simulink model "DK_KGTT"  (R2018a)
settings: Solver=VariableStepAuto  StartTime=0.0  StopTime=10.0  RelTol=1e-3
libraries: simulink x3
settings Model: Creator=dtan  LastModifiedBy=dtan

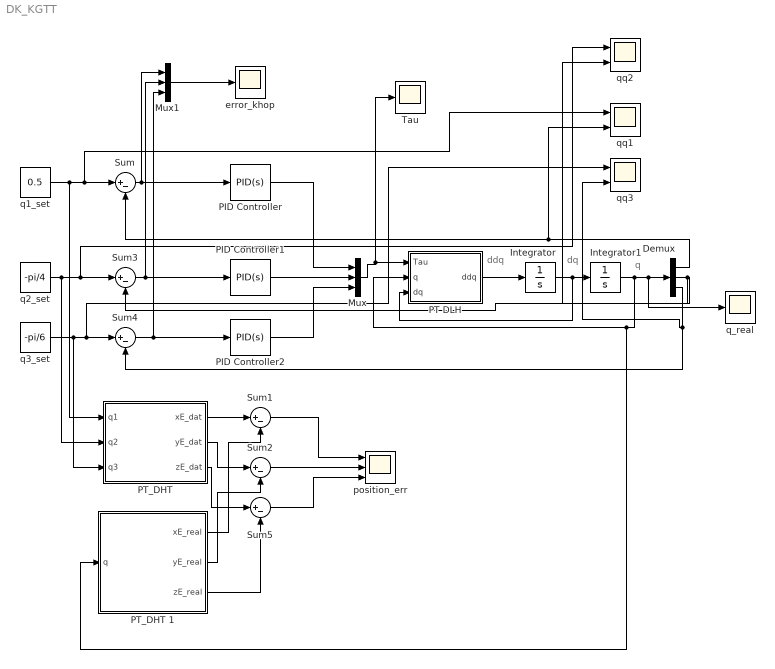
== system DK_KGTT ==
  note: q
  note: dq
  note: ddq
  Demux : Demux  Outputs=3
  Integrator : Integrator
  Integrator1 : Integrator
  Mux : Mux  Inputs=3
  Mux1 : Mux  Inputs=3
  PID Controller : simulink/Continuous/PID Controller  Controller=PID  TimeDomain=Continuous-time  SampleTime=-1  IntegratorMethod=Forward Euler  FilterMethod=Forward Euler  Form=Parallel  UseFilter=on  ControllerParametersSource=internal  P=50  I=30  D=10  N=100  InitialConditionSource=internal  InitialConditionForIntegrator=0  InitialConditionForFilter=0  ExternalReset=none  LimitOutput=off  UpperSaturationLimit=inf  LowerSaturationLimit=-inf  LinearizeAsGain=on  AntiWindupMode=none  Kb=1  TrackingMode=off  Kt=1  PParamMin=[]  PParamMax=[]  IParamMin=[]  IParamMax=[]  DParamMin=[]  DParamMax=[]  NParamMin=[]  NParamMax=[]  KbParamMin=[]  KbParamMax=[]  KtParamMin=[]  KtParamMax=[]  POutMin=[]  POutMax=[]  IOutMin=[]  IOutMax=[]  DOutMin=[]  DOutMax=[]  NOutMin=[]  NOutMax=[]  KbOutMin=[]  KbOutMax=[]  KtOutMin=[]  KtOutMax=[]  IntegratorOutMin=[]  IntegratorOutMax=[]  FilterOutMin=[]  FilterOutMax=[]  SumOutMin=[]  SumOutMax=[]  SumI1OutMin=[]  SumI1OutMax=[]  SumI2OutMin=[]  SumI2OutMax=[]  SumI3OutMin=[]  SumI3OutMax=[]  SumDOutMin=[]  SumDOutMax=[]  SaturationOutMin=[]  SaturationOutMax=[]  IntegratorContinuousStateAttributes=''  IntegratorStateMustResolveToSignalObject=off  IntegratorRTWStateStorageClass=Auto  FilterContinuousStateAttributes=''  FilterStateMustResolveToSignalObject=off  FilterRTWStateStorageClass=Auto  DifferentiatorICPrevScaledInput=0  DifferentiatorOutMin=[]  DifferentiatorOutMax=[]  FilterDiffOutCoefMin=[]  FilterDiffOutCoefMax=[]  SumDenOutMin=[]  SumDenOutMax=[]  SumNumOutMin=[]  SumNumOutMax=[]  ReciprocalOutMin=[]  ReciprocalOutMax=[]  DivideOutMin=[]  DivideOutMax=[]  TunerSelectOption=Transfer Function Based (PID Tuner App)
  PID Controller1 : simulink/Continuous/PID Controller  Controller=PID  TimeDomain=Continuous-time  SampleTime=-1  IntegratorMethod=Forward Euler  FilterMethod=Forward Euler  Form=Parallel  UseFilter=on  ControllerParametersSource=internal  P=20  I=0.2  D=0.8  N=100  InitialConditionSource=internal  InitialConditionForIntegrator=0  InitialConditionForFilter=0  ExternalReset=none  LimitOutput=off  UpperSaturationLimit=inf  LowerSaturationLimit=-inf  LinearizeAsGain=on  AntiWindupMode=none  Kb=1  TrackingMode=off  Kt=1  PParamMin=[]  PParamMax=[]  IParamMin=[]  IParamMax=[]  DParamMin=[]  DParamMax=[]  NParamMin=[]  NParamMax=[]  KbParamMin=[]  KbParamMax=[]  KtParamMin=[]  KtParamMax=[]  POutMin=[]  POutMax=[]  IOutMin=[]  IOutMax=[]  DOutMin=[]  DOutMax=[]  NOutMin=[]  NOutMax=[]  KbOutMin=[]  KbOutMax=[]  KtOutMin=[]  KtOutMax=[]  IntegratorOutMin=[]  IntegratorOutMax=[]  FilterOutMin=[]  FilterOutMax=[]  SumOutMin=[]  SumOutMax=[]  SumI1OutMin=[]  SumI1OutMax=[]  SumI2OutMin=[]  SumI2OutMax=[]  SumI3OutMin=[]  SumI3OutMax=[]  SumDOutMin=[]  SumDOutMax=[]  SaturationOutMin=[]  SaturationOutMax=[]  IntegratorContinuousStateAttributes=''  IntegratorStateMustResolveToSignalObject=off  IntegratorRTWStateStorageClass=Auto  FilterContinuousStateAttributes=''  FilterStateMustResolveToSignalObject=off  FilterRTWStateStorageClass=Auto  DifferentiatorICPrevScaledInput=0  DifferentiatorOutMin=[]  DifferentiatorOutMax=[]  FilterDiffOutCoefMin=[]  FilterDiffOutCoefMax=[]  SumDenOutMin=[]  SumDenOutMax=[]  SumNumOutMin=[]  SumNumOutMax=[]  ReciprocalOutMin=[]  ReciprocalOutMax=[]  DivideOutMin=[]  DivideOutMax=[]  TunerSelectOption=Transfer Function Based (PID Tuner App)
  PID Controller2 : simulink/Continuous/PID Controller  Controller=PID  TimeDomain=Continuous-time  SampleTime=-1  IntegratorMethod=Forward Euler  FilterMethod=Forward Euler  Form=Parallel  UseFilter=on  ControllerParametersSource=internal  P=50  I=30  D=10  N=100  InitialConditionSource=internal  InitialConditionForIntegrator=0  InitialConditionForFilter=0  ExternalReset=none  LimitOutput=off  UpperSaturationLimit=inf  LowerSaturationLimit=-inf  LinearizeAsGain=on  AntiWindupMode=none  Kb=1  TrackingMode=off  Kt=1  PParamMin=[]  PParamMax=[]  IParamMin=[]  IParamMax=[]  DParamMin=[]  DParamMax=[]  NParamMin=[]  NParamMax=[]  KbParamMin=[]  KbParamMax=[]  KtParamMin=[]  KtParamMax=[]  POutMin=[]  POutMax=[]  IOutMin=[]  IOutMax=[]  DOutMin=[]  DOutMax=[]  NOutMin=[]  NOutMax=[]  KbOutMin=[]  KbOutMax=[]  KtOutMin=[]  KtOutMax=[]  IntegratorOutMin=[]  IntegratorOutMax=[]  FilterOutMin=[]  FilterOutMax=[]  SumOutMin=[]  SumOutMax=[]  SumI1OutMin=[]  SumI1OutMax=[]  SumI2OutMin=[]  SumI2OutMax=[]  SumI3OutMin=[]  SumI3OutMax=[]  SumDOutMin=[]  SumDOutMax=[]  SaturationOutMin=[]  SaturationOutMax=[]  IntegratorContinuousStateAttributes=''  IntegratorStateMustResolveToSignalObject=off  IntegratorRTWStateStorageClass=Auto  FilterContinuousStateAttributes=''  FilterStateMustResolveToSignalObject=off  FilterRTWStateStorageClass=Auto  DifferentiatorICPrevScaledInput=0  DifferentiatorOutMin=[]  DifferentiatorOutMax=[]  FilterDiffOutCoefMin=[]  FilterDiffOutCoefMax=[]  SumDenOutMin=[]  SumDenOutMax=[]  SumNumOutMin=[]  SumNumOutMax=[]  ReciprocalOutMin=[]  ReciprocalOutMax=[]  DivideOutMin=[]  DivideOutMax=[]  TunerSelectOption=Transfer Function Based (PID Tuner App)
  PT DLH : MATLAB Function  TreatAsAtomicUnit=on
  "PT_DHT " : MATLAB Function  TreatAsAtomicUnit=on
  PT_DHT 1 : MATLAB Function  TreatAsAtomicUnit=on
  Sum{,1..5} (6 alike) : Sum  Inputs=|+-
  "Tau " : Scope
  "error_khop " : Scope
  position_err : Scope  NumInputPorts=3
  "q1_set " : Constant  Value=0.5
  q2_set : Constant  Value=-pi/4
  "q3_set " : Constant  Value=-pi/6
  "q_real " : Scope
  qq1 : Scope  NumInputPorts=2
  qq2 : Scope  NumInputPorts=2
  qq3 : Scope  NumInputPorts=2
  wires:
  Sum3/1 -> Mux1/2, PID Controller1/1
  PID Controller/1 -> Mux/1
  Demux/3 -> qq3/2, Sum4/2
  Demux/2 -> qq2/2, Sum3/2
  Mux/1 -> "Tau "/1, PT DLH/1(Tau)
  q2_set/1 -> "PT_DHT "/2(q2), qq2/1, Sum3/1
  Integrator1/1 -> "q_real "/1, Demux/1, PT_DHT 1/1(q), PT DLH/2(q)
  PID Controller1/1 -> Mux/2
  Integrator/1 -> PT DLH/3(dq), Integrator1/1
  "q1_set "/1 -> "PT_DHT "/1(q1), qq1/1, Sum/1
  Demux/1 -> qq1/2, Sum/2
  Sum4/1 -> Mux1/3, PID Controller2/1
  Mux1/1 -> "error_khop "/1
  PID Controller2/1 -> Mux/3
  PT DLH/1(ddq) -> Integrator/1
  "q3_set "/1 -> "PT_DHT "/3(q3), qq3/1, Sum4/1
  Sum/1 -> PID Controller/1, Mux1/1
  "PT_DHT "/1(xE_dat) -> Sum1/1
  PT_DHT 1/1(xE_real) -> Sum1/2
  "PT_DHT "/2(yE_dat) -> Sum2/1
  PT_DHT 1/2(yE_real) -> Sum2/2
  "PT_DHT "/3(zE_dat) -> Sum5/1
  PT_DHT 1/3(zE_real) -> Sum5/2
  Sum1/1 -> position_err/1
  Sum2/1 -> position_err/2
  Sum5/1 -> position_err/3

== matlab function DK_KGTT/PT DLH ==
  data: Tau input; q input; dq input; ddq output
function ddq =DLH(Tau,q,dq)
[m1,m2,m3,L1,L2,L3,I1x,I1y,I1z,I2x,I2y,I2z,I3x,I3y,I3z]=parameter3DOF()
q = zeros(3,1);
dq = zeros(3,1);
% Khai bao ma tran khoi luong M
M=zeros(3,3);
M(1,1)= m1+m2+m3;
M(1,2)= -(1/2)*m2*cos(q(2))*L2-(3/2)*m3*sin(q(2))*L3*cos(q(3));
M(1,3)= -(3/2)*m3*cos(q(2))*L3*sin(q(3));


M(2,1)=-(1/2)*m2*cos(q(2))*L2-(3/2)*m3*sin(q(2))*L3*cos(q(3));
M(2,2)=(1/4)*m2*L2^2+I2y+(9/4)*m3*L3^2*cos(q(3))^2-I3x*cos(q(3))^2+cos(q(3))^2*I3y+I3x;
M(2,3)=0;

M(3,1)=-(3/2)*m3*cos(q(2))*L3*sin(q(3));
M(3,2)=0;
M(3,3)=(9/4)*m3*L3^2+I3z;

% Khai bao ma tran Coriolis C
%h=-m2*L1*Lc2*sin(q(2));
Co=zeros(3,3);
Co(1,1)=0;
Co(1,2)=-(3/2)*dq(2)*m3*cos(q(2))*L3*cos(q(3))+(3/2)*m3*sin(q(2))*L3*sin(q(3))*dq(3)+(1/2)*dq(2)*m2*sin(q(2))*L2;
Co(1,3)=-(3/2)*m3*L3*(dq(3)*cos(q(2))*cos(q(3))-dq(2)*sin(q(2))*sin(q(3)));


Co(2,1)=-(3/4)*dq(2)*m3*cos(q(2))*L3*cos(q(3))+(3/4)*m3*sin(q(2))*L3*sin(q(3))*dq(3)+(1/4)*dq(2)*m2*sin(q(2))*L2;
Co(2,2)=-(9/2)*L3^2*cos(q(3))*sin(q(3))*dq(3)*m3+(3/4)*m3*cos(q(2))*L3*cos(q(3))*dq(1)+2*I3x*cos(q(3))*sin(q(3))*dq(3)-2*I3y*cos(q(3))*sin(q(3))*dq(3)-(1/4)*dq(1)*m2*sin(q(2))*L2;
Co(2,3)=-(3/4)*m3*sin(q(2))*L3*sin(q(3))*dq(1);


Co(3,1)=-(3/4)*m3*L3*(dq(3)*cos(q(2))*cos(q(3))-dq(2)*sin(q(2))*sin(q(3)));
Co(3,2)=-(1/4)*sin(q(3))*(-9*L3^2*cos(q(3))*dq(2)*m3+3*m3*sin(q(2))*L3*dq(1)+4*I3x*cos(q(3))*dq(2)-4*I3y*cos(q(3))*dq(2));
Co(3,3)=(3/4)*m3*cos(q(2))*L3*cos(q(3))*dq(1);

% Ma tran the nang hap dan
G=zeros(3,1);
G(1,1)=0;
G(2,1)=0;
G(3,1)=-15*m3*L3*cos(q(3));


% Pt DLH
ddq = inv(M)*(Tau - Co*dq -G);

== matlab function DK_KGTT/PT_DHT  ==
  data: q1 input; xE_dat output; q2 input; q3 input; yE_dat output; zE_dat output
function [xE_dat,yE_dat,zE_dat] = DHT(q1,q2,q3)
[m1,m2,m3,L1,L2,L3,I1x,I1y,I1z,I2x,I2y,I2z,I3x,I3y,I3z]=parameter3DOF();
xE_dat= cos(q2)*L3*cos(q3)+q1;
yE_dat= sin(q2)*L3*cos(q3);
zE_dat= -L3*sin(q3)+L2;
end

== matlab function DK_KGTT/PT_DHT 1 ==
  data: q input; xE_real output; yE_real output; zE_real output
function [xE_real,yE_real,zE_real] = DHT(q)
[m1,m2,m3,L1,L2,L3,I1x,I1y,I1z,I2x,I2y,I2z,I3x,I3y,I3z]=parameter3DOF();
xE_real= cos(q(2))*L3*cos(q(3))+q(1);
yE_real= sin(q(2))*L3*cos(q(3));
zE_real= -L3*sin(q(3))+L2;
end
